simulink library "dbdc"  (Simulink 8.1)
settings: Solver=ode1  StartTime=0.0  StopTime=Inf  FixedStep=0.001  RelTol=1e-3
PostLoadFcn:
  | , if any(exist('dsrtsu_mdlpostloadfcn', 'file') == [2, 3, 6]), try dsrtsu_mdlpostloadfcn('Execute', bdroot); catch fprintf('Error in PostLoadFcn (dsrtsu_mdlpostloadfcn) for model "%s":\n %s\n', bdroot, lasterr); end, end,
undefined symbols (not defined in the file or in its folder): KJUD_FCWActiveDriverDelay_ms, KJUD_FCWAggrDriverDelay_ms, ZERO_FLOAT
settings Model: DSRTSU_INTERNAL_RTI_VER=450  DSRTSU_INTERNAL_RTI_TYPE=rti1401  Creator=idiada  LastModifiedBy=idiada

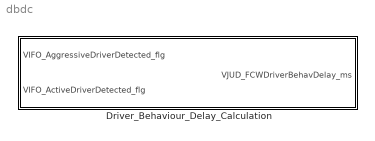
== system dbdc ==
  Driver_Behaviour_Delay_Calculation : Subsystem

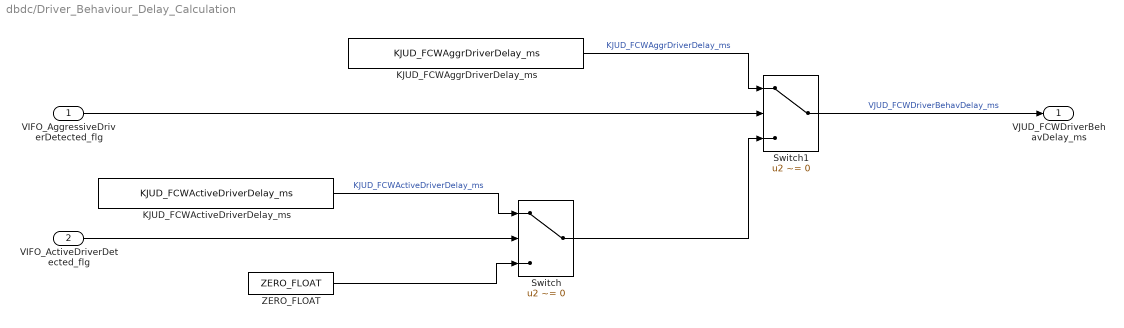
== system dbdc/Driver_Behaviour_Delay_Calculation ==
  VIFO_AggressiveDriverDetected_flg : Inport
  VIFO_ActiveDriverDetected_flg : Inport  Port=2
  KJUD_FCWActiveDriverDelay_ms : Constant  Value=KJUD_FCWActiveDriverDelay_ms  OutDataTypeStr=single
  KJUD_FCWAggrDriverDelay_ms : Constant  Value=KJUD_FCWAggrDriverDelay_ms  OutDataTypeStr=single
  Switch : Switch  Criteria=u2 ~= 0
  Switch1 : Switch  Criteria=u2 ~= 0
  ZERO_FLOAT : Constant  Value=ZERO_FLOAT  OutDataTypeStr=single
  VJUD_FCWDriverBehavDelay_ms : Outport
  wires:
  VIFO_ActiveDriverDetected_flg/1 -> Switch/2
  Switch1/1 -> VJUD_FCWDriverBehavDelay_ms/1  "VJUD_FCWDriverBehavDelay_ms"
  ZERO_FLOAT/1 -> Switch/3
  KJUD_FCWActiveDriverDelay_ms/1 -> Switch/1  "KJUD_FCWActiveDriverDelay_ms"
  VIFO_AggressiveDriverDetected_flg/1 -> Switch1/2
  Switch/1 -> Switch1/3
  KJUD_FCWAggrDriverDelay_ms/1 -> Switch1/1  "KJUD_FCWAggrDriverDelay_ms"
